simulink model "E030_C4_pisiek_proj_iqcot_20260629"  (R2024b)
settings: Solver=VariableStepAuto  StartTime=0.0  StopTime=0.64e-3  MaxStep=5e-9  RelTol=1e-3
undefined symbols (not defined in the file): A_init, A_lower, A_upper, Cout, DCR_L1, DCR_L2, DCR_L3, DCR_L4, E030_Current_Deadband, E030_K_Lambda, E030_K_T, E030_Lambda_Trim_Max, E030_LambdaDiff_Enable, E030_Nominal_Phase_Spacing, E030_Phase_Spacing_Tolerance, E030_PIS_Project_Enable, E030_T_Trim_Max, E030_TonDiff_Enable, ESR_C, IdealIQCOT_Enable, IL_adc_counts_per_A, IL_pk_limit_adc_neg, IL_pk_limit_adc_pos, Iload_final, Iload_initial, Iph, Iqcot_enable, kappa_cmd, Kiqcot, Kvc_iqcot, L, Lambda0_iqcot, Lambda_m2, rho_cmd, Ri_iqcot, t_load_step, Tblank, Tdead, Tiqcot_leak, Toff_min, Ton_cmd, Ton_iq_max, Ton_iq_min, Ts_ctrl, Tslot, Tss, Vc_bias_iqcot, Vcot_ramp_amp, Vcot_ramp_enable, Vhys, Vin, Vo_ref
libraries: simulink x29, spsCurrentMeasurementLib x8, spsMosfetLib x8, spsSeriesRLCBranchLib x5, spsVoltageMeasurementLib x5, spsDCVoltageSourceLib x4, spsControlledCurrentSourceLib x1, spsGroundLib x1, spspowerguiLib x1
(part 2 of 2)

== matlab function E030_C4_pisiek_proj_iqcot_20260629/E030_LambdaDiff_Controller ==
  data: tr1 input boolean size=1; tr1o output boolean size=1; tr2 input boolean size=1; tr3 input boolean size=1; tr4 input boolean size=1; t input double size=1; enable input double size=1; nominal_spacing input double size=1; tolerance input double size=1; lambda_max input double size=1; K_lambda input double size=1; projected input double size=1; tr2o output boolean size=1; tr3o output boolean size=1; tr4o output boolean size=1; lam1 output double size=1; lam2 output double size=1; lam3 output double size=1; lam4 output double size=1; clamp_count output double size=1; fallback_count output double size=1
function [tr1o,tr2o,tr3o,tr4o,lam1,lam2,lam3,lam4,clamp_count,fallback_count] = lambda_diff(tr1,tr2,tr3,tr4,t,enable,nominal_spacing,tolerance,lambda_max,K_lambda,projected)
%#codegen
persistent last_any
if isempty(last_any)
    last_any = -1.0;
end
tr = [logical(tr1), logical(tr2), logical(tr3), logical(tr4)];
out = tr;
trim = zeros(1,4);
clamp_count = 0.0;
fallback_count = 0.0;
if enable > 0.5
    for idx = 1:4
        if tr(idx)
            if last_any < 0.0
                spacing = nominal_spacing;
            else
                spacing = t - last_any;
            end
            err = spacing - nominal_spacing;
            raw = -K_lambda * err;
            trim(idx) = min(max(raw, -lambda_max), lambda_max);
            if abs(raw) > lambda_max || abs(err) > tolerance
                clamp_count = clamp_count + 1.0;
            end
            last_any = t;
        end
    end
    trim = trim - mean(trim);
    if projected > 0.5 && clamp_count > 0.5
        trim = zeros(1,4);
        fallback_count = 1.0;
    end
else
    for idx = 1:4
        if tr(idx)
            last_any = t;
        end
    end
end
tr1o = out(1); tr2o = out(2); tr3o = out(3); tr4o = out(4);
lam1 = trim(1); lam2 = trim(2); lam3 = trim(3); lam4 = trim(4);

== matlab function E030_C4_pisiek_proj_iqcot_20260629/Ideal_Digital_IQCOT_Request/IQCOT_Event_Core ==
  data: e_v input double size=1; REQ_iqcot output double size=1; IL1 input double size=1; IL2 input double size=1; IL3 input double size=1; IL4 input double size=1; phase_idx input double size=1; tr_reset input double size=1; enable input double size=1; Ts_ctrl_in input double size=1; Lambda0_in input double size=1; Lambda_m2_in input double size=1; rho_cmd_in input double size=1; Ri_in input double size=1; Kvc_in input double size=1; Vc_bias_in input double size=1; kappa_cmd_in input double size=1; A_init_in input double size=1; A_lower_in input double size=1; A_upper_in input double size=1; A_iqcot output double size=1; Lambda_i output double size=1; h_iqcot output double size=1; IL_sel output double size=1; vc_ctrl output double size=1
function [REQ_iqcot,A_iqcot,Lambda_i,h_iqcot,IL_sel,vc_ctrl] = IQCOT_Event_Core(e_v,IL1,IL2,IL3,IL4,phase_idx,tr_reset,enable,Ts_ctrl_in,Lambda0_in,Lambda_m2_in,rho_cmd_in,Ri_in,Kvc_in,Vc_bias_in,kappa_cmd_in,A_init_in,A_lower_in,A_upper_in)
%#codegen
REQ_iqcot = 0.0;
A_iqcot = 0.0;
Lambda_i = 0.0;
h_iqcot = 0.0;
IL_sel = 0.0;
vc_ctrl = 0.0;
persistent Astate reset_prev phase_prev
if isempty(Astate)
    Astate = double(A_init_in);
end
if isempty(reset_prev)
    reset_prev = 0.0;
end
if isempty(phase_prev)
    phase_prev = 0.0;
end
p = floor(double(phase_idx));
p = mod(p, 4);
if p == 0
    IL_sel = IL1;
elseif p == 1
    IL_sel = IL2;
elseif p == 2
    IL_sel = IL3;
else
    IL_sel = IL4;
end
Ri_eff = Ri_in * exp(kappa_cmd_in);
vc_ctrl = Vc_bias_in + Kvc_in * e_v;
h_iqcot = vc_ctrl - Ri_eff * IL_sel;
Lambda_i = Lambda0_in * (1 + rho_cmd_in) + Lambda_m2_in * cos(pi * p);
if Lambda_i < eps
    Lambda_i = eps;
end
A_update = Astate + Ts_ctrl_in * h_iqcot;
if A_update < A_lower_in
    A_update = A_lower_in;
end
if A_update > A_upper_in
    A_update = A_upper_in;
end
REQ_iqcot = double((enable > 0.5) && (A_update >= Lambda_i));
A_iqcot = A_update;
reset_rise = (tr_reset > 0.5) && (reset_prev <= 0.5);
phase_change = (p ~= phase_prev);
if enable <= 0.5
    Astate = A_init_in;
elseif reset_rise || phase_change
    Astate = A_init_in;
else
    Astate = A_update;
end
reset_prev = double(tr_reset);
phase_prev = p;

== matlab function E030_C4_pisiek_proj_iqcot_20260629/E030_TonDiff_Controller ==
  data: ton1 input double size=1; ton1o output double size=1; ton2 input double size=1; ton3 input double size=1; ton4 input double size=1; il1 input double size=1; il2 input double size=1; il3 input double size=1; il4 input double size=1; enable input double size=1; K_T input double size=1; T_trim_max input double size=1; deadband input double size=1; projected input double size=1; ton2o output double size=1; ton3o output double size=1; ton4o output double size=1; trim1 output double size=1; trim2 output double size=1; trim3 output double size=1; trim4 output double size=1; clamp_count output double size=1; fallback_count output double size=1
function [ton1o,ton2o,ton3o,ton4o,trim1,trim2,trim3,trim4,clamp_count,fallback_count] = ton_diff(ton1,ton2,ton3,ton4,il1,il2,il3,il4,enable,K_T,T_trim_max,deadband,projected)
%#codegen
tons = [ton1, ton2, ton3, ton4];
ils = [il1, il2, il3, il4];
avg = mean(ils);
err = ils - avg;
raw = -K_T .* err;
if enable <= 0.5
    trim = zeros(1,4);
    clamp_count = 0.0;
    fallback_count = 0.0;
else
    if projected > 0.5 && max(abs(err)) < deadband
        raw = zeros(1,4);
    end
    trim = min(max(raw, -T_trim_max), T_trim_max);
    clamp_count = double(any(abs(raw) > T_trim_max));
    trim = trim - mean(trim);
    fallback_count = 0.0;
end
outs = max(0.0, tons + trim);
ton1o = outs(1); ton2o = outs(2); ton3o = outs(3); ton4o = outs(4);
trim1 = trim(1); trim2 = trim(2); trim3 = trim(3); trim4 = trim(4);
